simulink model "Robot_Sim_bkp2"  (R2017a)
settings: Solver=VariableStepAuto  StartTime=0.0  StopTime=Tsim  FixedStep=Ts_compute  RelTol=1e-3
values from neighbouring files (symbols this model uses):
  b = 0.1    [Model_old.m]
  g = 40    [Model_old.m]    (also in ModeloBase_OLD.m)
  Gyro_bias = 0.004    [Model_old.m]
  Kd = 0    [Model_old.m]
  Ki = 10.0    (= 10)    [Model_old.m]
  Kp = 5.0    (= 5)    [Model_old.m]
  ksi = 0.6    [Model_old.m]    (also in ModeloBase_OLD.m = 0.3)
  Ts = 0.1    [Model_old.m]    (also in ModeloBase_OLD.m; PIController.m)
  Ts_sensor = 1/50    (= 0.02)    [Model_old.m]
  Tsim = 50    [Model_old.m]    (also in ModeloBase_OLD.m = 70)
undefined symbols (not defined in the file or in its folder): Aa, Ag, Ba, Bg, Ca, Cg, DiscIntNeverNeededParam, Discrete, K_KALM_g, K_LQ, Rna, Rng, Time, W
undefined symbols (not defined in the file): Qna
libraries: simulink x13, ctrlSharedLib x2, cstblocks x2
settings Model: PauseTimes=28  NumberOfSteps=10  Creator=davi2  LastModifiedBy=marcus

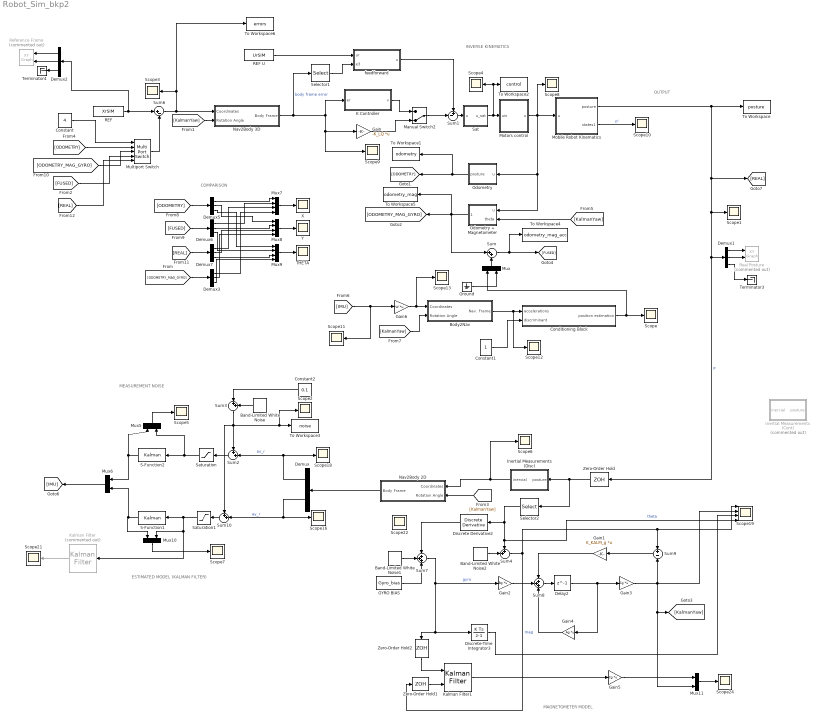
== system Robot_Sim_bkp2 ==
  note: COMPARISON
  note: OUTPUT
  note: MEASUREMENT NOISE
  note: INVERSE KINEMATICS
  note: MAGNETOMETER MODEL
  note: ESTIMATED MODEL (KALMAN FILTER)
  Band-Limited White Noise : simulink/Sources/Band-Limited White Noise  Cov=Rna^2  Ts=Ts_sensor  seed=[23341]
  Band-Limited White Noise1 : simulink/Sources/Band-Limited White Noise  Cov=0.00001  Ts=Ts_sensor  seed=[23341]
  Band-Limited White Noise2 : simulink/Sources/Band-Limited White Noise  Cov=Rng^2  Ts=Ts_sensor  seed=[23341]
  Body2Nav : Subsystem
  Conditioning Block : Subsystem
  Constant : Constant  Value=4
  Constant1 : Constant
  Constant2 : Constant  Value=0.1
  Delay2 : Delay  DelayLength=1
  Demux : Demux  Outputs=2
  Demux{1..3,5..7} (6 alike) : Demux  Outputs=3
  Discrete Derivative2 : simulink/Discrete/Discrete Derivative  gainval=1.0  ICPrevScaledInput=0.0  OutMin=[]  OutMax=[]  OutDataType=fixdt(1, 16)  OutScaling=2^-10  DoSatur=off
  Discrete-Time Integrator3 : DiscreteIntegrator  InitialConditionSetting=State (most efficient)  SampleTime=-1  ICPrevOutput=DiscIntNeverNeededParam  ICPrevScaledInput=DiscIntNeverNeededParam
  GYRO BIAS : Constant  Value=Gyro_bias
  Gain : Gain  Gain=-K_LQ  Multiplication=Matrix(K*u)
  Gain1 : Gain  Gain=K_KALM_g  Multiplication=Matrix(K*u)
  Gain2 : Gain  Gain=Bg  Multiplication=Matrix(K*u)
  Gain3 : Gain  Gain=Cg  Multiplication=Matrix(K*u)
  Gain4 : Gain  Gain=Ag  Multiplication=Matrix(K*u)
  Gain5 : Gain  Gain=Cg  Multiplication=Matrix(K*u)
  Gain6 : Gain  Gain=W  Multiplication=Matrix(K*u)
  Ground : Ground
  Inertial Measurements (Cont) : Subsystem  Commented=on
  Inertial Measurements (Disc) : Subsystem
  K Controller : Subsystem
  Kalman Filter : ctrlSharedLib/Kalman Filter  Commented=on  TimeDomain=Discrete-Time  UseCurrentEstimator=on  ModelSource=LTI State-Space Variable  ModelSourceVariable=ss(Aa,Ba,Ca,0,Ts_sensor)  A=0.95  B=1  C=1  D=0  NumberOfStates=1  NumberOfInputs=1  NumberOfOutputs=1  InitialEstimateSource=Dialog  X0=0  P0=10  UseK=off  UseGH=off  NumberOfProcessNoiseInputs=1  G=1  TimeInvariantG=on  H=0  TimeInvariantH=on  Q=Qna  TimeInvariantQ=on  R=Rna  TimeInvariantR=on  N=0  TimeInvariantN=on  AddInputPort=off  AddEnablePort=off  OutputEstimatedY=off  OutputP=off  Ts=-1
  Kalman Filter1 : ctrlSharedLib/Kalman Filter  TimeDomain=Discrete-Time  UseCurrentEstimator=on  ModelSource=LTI State-Space Variable  ModelSourceVariable=ss(Ag,Bg,Cg,0,Ts_sensor)  A=0.95  B=1  C=1  D=0  NumberOfStates=1  NumberOfInputs=1  NumberOfOutputs=1  InitialEstimateSource=Dialog  X0=0  P0=10  UseK=off  UseGH=off  NumberOfProcessNoiseInputs=1  G=1  TimeInvariantG=on  H=0  TimeInvariantH=on  Q=Qng  TimeInvariantQ=on  R=Rng  TimeInvariantR=on  N=0  TimeInvariantN=on  AddInputPort=on  AddEnablePort=off  OutputEstimatedY=off  OutputP=off  Ts=-1
  Manual Switch2 : ManualSwitch  CurrentSetting=0
  Mobile Robot Kinematics : Subsystem
  Motors control : Subsystem
  Multiport Switch : MultiPortSwitch  Inputs=4
  Mux{,5..6,10..11} (5 alike) : Mux  Inputs=2
  Mux7 : Mux
  Mux8 : Mux
  Mux9 : Mux
  Nav2Body 2D : Subsystem
  Nav2Body 3D : Subsystem
  Odometry : Subsystem
  Odometry + Magnetometer : Subsystem
  REF : FromWorkspace  VariableName=XrSIM  SampleTime=Ts  OutputAfterFinalValue=Holding final value
  REF U : FromWorkspace  VariableName=UrSIM  SampleTime=Ts  OutputAfterFinalValue=Holding final value
  Real Posture : simulink/Sinks/XY Graph  Commented=on  xmin=0  xmax=3  ymin=-0.8  ymax=1.5  st=Ts
  Reference Frame : simulink/Sinks/XY Graph  Commented=on  xmin=0  xmax=2  ymin=0  ymax=1.5  st=Ts
  S-Function1 : S-Function  FunctionName=Kalman  Parameters=Ts_sensor,A,C,Rw,Rv  SFunctionDeploymentMode=off  EnableBusSupport=off  mask{Ts=Ts_sensor, A=Aa, C=Ca, Rv=Rna, Rw=Qna}
      mask prompts: Ts "Tempo de Amostragem"; A "Matriz A"; C "Matriz C"; Rv "Covariancia da Saida"; Rw "Covariancia do Processo"
      mask DialogControl DescTextVar Tooltip: Filtro
      mask Display: disp('MyKalman')
  S-Function2 : S-Function  FunctionName=Kalman  Parameters=Ts_sensor,A,C,Rw,Rv  SFunctionDeploymentMode=off  EnableBusSupport=off  mask{Ts=Ts_sensor, A=Aa, C=Ca, Rv=Rna, Rw=Qna}
      mask prompts: Ts "Tempo de Amostragem"; A "Matriz A"; C "Matriz C"; Rv "Covariancia da Saida"; Rw "Covariancia do Processo"
      mask DialogControl DescTextVar Tooltip: Filtro
      mask Display: disp('MyKalman')
  Sat : Subsystem
  Saturation : Saturate  UpperLimit=4*9.8  LowerLimit=-4*9.8
  Saturation1 : Saturate  UpperLimit=4*9.8  LowerLimit=-4*9.8
  Scope{,1..13,16,18,21..22,24} (19 alike) : Scope
  Scope19 : Scope  NumInputPorts=4
  Selector1 : Selector  InputPortWidth=3  IndexOptions=Index vector (dialog)  Indices=3  OutputSizes=1
  Selector2 : Selector  InputPortWidth=3  IndexOptions=Index vector (dialog)  Indices=3  OutputSizes=1
  Sum : Sum  Inputs=|++
  Sum1 : Sum  Inputs=+-|
  Sum10 : Sum  Inputs=++|
  Sum2 : Sum  Inputs=++|
  Sum3 : Sum  Inputs=|++
  Sum4 : Sum  Inputs=++|
  Sum6 : Sum  Inputs=|+-
  Sum7 : Sum  Inputs=+++
  Sum8 : Sum  Inputs=+++
  Sum9 : Sum  Inputs=+-
  THETA : Scope
  Terminator3 : Terminator
  Terminator4 : Terminator
  To Workspace : ToWorkspace  VariableName=posture  SaveFormat=Timeseries  SampleTime=-1
  To Workspace1 : ToWorkspace  VariableName=odometry  SaveFormat=Timeseries  SampleTime=-1
  To Workspace2 : ToWorkspace  VariableName=control  SaveFormat=Timeseries  SampleTime=-1
  To Workspace3 : ToWorkspace  VariableName=noise  SaveFormat=Timeseries  SampleTime=-1
  To Workspace4 : ToWorkspace  VariableName=odometry_mag_acc  SaveFormat=Timeseries  SampleTime=-1
  To Workspace5 : ToWorkspace  VariableName=odometry_mag  SaveFormat=Timeseries  SampleTime=-1
  To Workspace6 : ToWorkspace  VariableName=errors  SaveFormat=Timeseries  SampleTime=-1
  X : Scope
  Y : Scope
  Zero-Order Hold : ZeroOrderHold  SampleTime=Ts_sensor
  Zero-Order Hold1 : ZeroOrderHold  SampleTime=Ts_sensor
  Zero-Order Hold2 : ZeroOrderHold  SampleTime=Ts_sensor
  feedforward : Subsystem
  wires:
  Nav2Body 3D/1(Body Frame) -> Scope9/1, Gain/1, K Controller/1(er), Selector1/1  "body frame error"
  REF U/1 -> feedforward/1(ur)
  Selector1/1 -> feedforward/2(e3)
  Motors control/1(u) -> Odometry + Magnetometer/1(u), Odometry/1(u), Mobile Robot Kinematics/1(u), Scope8/1
  Selector2/1 -> Scope19/4, Sum4/1, Discrete Derivative2/1  "theta"
  Demux1/1 -> Real Posture/1
  Demux1/2 -> Real Posture/2
  Odometry/1(posture) -> To Workspace1/1, [ODOMETRY]
  Sum1/1 -> Sat/1(u)
  Sat/1(u_sat) -> Motors control/1(uin), Scope4/1, To Workspace2/1
  Demux1/3 -> Terminator3/1
  Band-Limited White Noise2/1 -> Sum4/2
  Demux2/1 -> Reference Frame/1
  Demux2/2 -> Reference Frame/2
  Demux2/3 -> Terminator4/1
  Mobile Robot Kinematics/1(posture) -> [REAL], Zero-Order Hold/1, Demux1/1, Scope1/1, To Workspace/1  "P"
  Demux/1 -> Scope18/1, Sum2/2  "ax_r"
  Demux/2 -> Sum10/2, Scope16/1  "ay_r"
  Inertial Measurements (Disc)/1(inercial) -> Scope6/1, Nav2Body 2D/1(Coordinates)
  REF/1 -> Sum6/1, Demux2/1
  Mux5/1 -> Scope5/1
  [KalmanYaw] -> Nav2Body 2D/2(Rotation Angle)
  Odometry + Magnetometer/1(posture) -> Sum/1, To Workspace5/1, [ODOMETRY_MAG_GYRO]
  [KalmanYaw] -> Odometry + Magnetometer/2(theta)
  [ODOMETRY] -> Demux5/1
  [FUSED] -> Demux6/1
  [REAL] -> Demux7/1
  Demux5/1 -> Mux7/1
  Demux6/1 -> Mux7/2
  Demux7/1 -> Mux7/3
  Mux7/1 -> X/1
  Demux5/2 -> Mux8/1
  Demux6/2 -> Mux8/2
  Demux7/2 -> Mux8/3
  Demux5/3 -> Mux9/1
  Demux6/3 -> Mux9/2
  Demux7/3 -> Mux9/3
  Mux8/1 -> Y/1
  Mux9/1 -> THETA/1
  Mobile Robot Kinematics/2(states1) -> Scope10/1  "p'"
  Sum3/1 -> Sum10/1, Sum2/1, Scope2/1, To Workspace3/1
  Band-Limited White Noise/1 -> Sum3/2
  Constant2/1 -> Sum3/1
  Sum10/1 -> Saturation1/1
  Sum2/1 -> Saturation/1
  Saturation1/1 -> S-Function1/1, Mux10/2, Kalman Filter/1
  Saturation/1 -> S-Function2/1, Mux5/2
  Mux10/1 -> Scope7/1
  S-Function1/1 -> Mux6/2, Mux10/1
  S-Function2/1 -> Mux6/1, Mux5/1
  Band-Limited White Noise1/1 -> Sum7/2
  Discrete Derivative2/1 -> Sum7/1
  GYRO BIAS/1 -> Sum7/3
  Sum7/1 -> Gain2/1, Discrete-Time Integrator3/1, Zero-Order Hold2/1  "gyro"
  Sum4/1 -> Scope19/1, Sum9/1, Zero-Order Hold1/1  "mag"
  Sum8/1 -> Delay2/1
  Gain2/1 -> Sum8/2
  Delay2/1 -> Gain3/1, Gain4/1
  Gain4/1 -> Sum8/3
  Gain1/1 -> Sum8/1
  Gain3/1 -> Scope19/2, Mux11/2, [KalmanYaw], Sum9/2
  Sum9/1 -> Gain1/1
  Discrete-Time Integrator3/1 -> Scope19/3
  Manual Switch2/1 -> Sum1/2
  feedforward/1(u) -> Sum1/1
  Gain/1 -> Manual Switch2/2
  K Controller/1(v) -> Manual Switch2/1
  Nav2Body 2D/1(Body Frame) -> Demux/1
  [KalmanYaw] -> Nav2Body 3D/2(Rotation Angle)
  Mux6/1 -> [IMU]
  Sum6/1 -> To Workspace6/1, Scope3/1, Nav2Body 3D/1(Coordinates)
  Kalman Filter/1 -> Scope21/1
  Zero-Order Hold1/1 -> Kalman Filter1/2
  Zero-Order Hold2/1 -> Kalman Filter1/1
  Kalman Filter1/1 -> Gain5/1
  Mux11/1 -> Scope24/1
  Gain5/1 -> Mux11/1
  Zero-Order Hold/1 -> Inertial Measurements (Disc)/1(posture), Selector2/1
  [ODOMETRY_MAG_GYRO] -> Demux3/1
  Demux3/1 -> Mux7/4
  Demux3/2 -> Mux8/4
  Demux3/3 -> Mux9/4
  [ODOMETRY] -> Multiport Switch/2
  [ODOMETRY_MAG_GYRO] -> Multiport Switch/3
  [FUSED] -> Multiport Switch/4
  Multiport Switch/1 -> Sum6/2
  Constant/1 -> Multiport Switch/1
  [KalmanYaw] -> Body2Nav/2(Rotation Angle)
  Sum/1 -> To Workspace4/1, [FUSED]
  Mux/1 -> Sum/2
  Ground/1 -> Mux/2
  Constant1/1 -> Conditioning Block/2(discriminant)
  [IMU] -> Gain6/1, Scope11/1
  Conditioning Block/1(position estimation) -> Mux/1, Scope/1
  [REAL] -> Multiport Switch/5
  Body2Nav/1(Nav. Frame) -> Scope12/1, Conditioning Block/1(accelerations)
  Gain6/1 -> Scope13/1, Body2Nav/1(Coordinates)

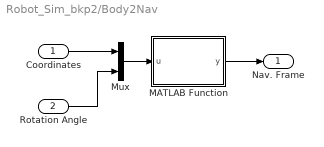
== system Robot_Sim_bkp2/Body2Nav ==
  Coordinates : Inport
  Rotation Angle : Inport  Port=2
  MATLAB Function : MATLAB Function  TreatAsAtomicUnit=on
  Mux : Mux  Inputs=2
  Nav. Frame : Outport
  wires:
  Coordinates/1 -> Mux/1
  Rotation Angle/1 -> Mux/2
  Mux/1 -> MATLAB Function/1(u)
  MATLAB Function/1(y) -> Nav. Frame/1

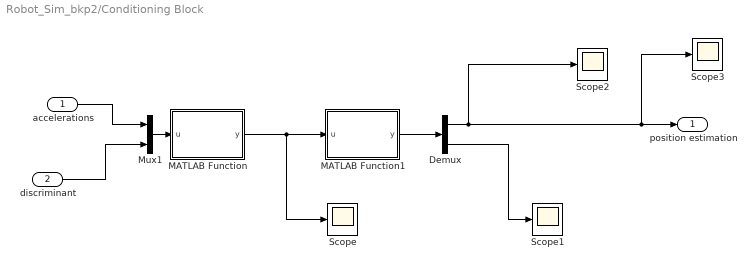
== system Robot_Sim_bkp2/Conditioning Block ==
  accelerations : Inport
  discriminant : Inport  Port=2
  Demux : Demux  Outputs=2
  MATLAB Function : MATLAB Function  TreatAsAtomicUnit=on
  MATLAB Function1 : MATLAB Function  TreatAsAtomicUnit=on
  Mux1 : Mux  Inputs=2
  Scope{,1..3} (4 alike) : Scope
  position estimation : Outport
  wires:
  Mux1/1 -> MATLAB Function/1(u)
  accelerations/1 -> Mux1/1
  MATLAB Function/1(y) -> MATLAB Function1/1(u), Scope/1
  MATLAB Function1/1(y) -> Demux/1
  discriminant/1 -> Mux1/2
  Demux/2 -> Scope1/1
  Demux/1 -> Scope3/1, position estimation/1, Scope2/1

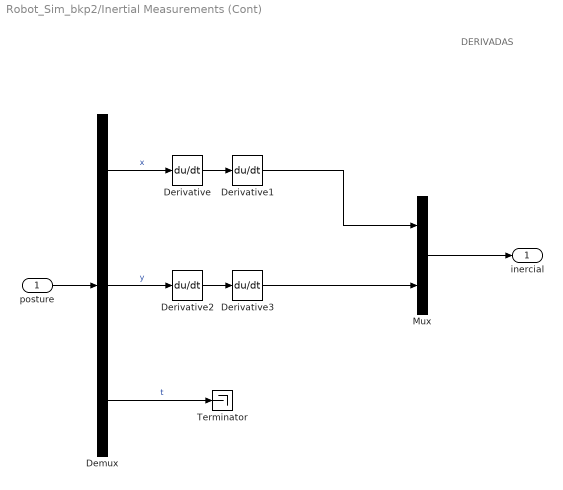
== system Robot_Sim_bkp2/Inertial Measurements (Cont) ==
  note: DERIVADAS
  posture : Inport
  Demux : Demux  Outputs=3
  Derivative{,1..3} (4 alike) : Derivative
  Mux : Mux  Inputs=2
  Terminator : Terminator
  inercial : Outport
  wires:
  posture/1 -> Demux/1
  Mux/1 -> inercial/1
  Demux/3 -> Terminator/1  "t"
  Derivative3/1 -> Mux/2
  Derivative1/1 -> Mux/1
  Demux/1 -> Derivative/1  "x"
  Demux/2 -> Derivative2/1  "y"
  Derivative/1 -> Derivative1/1
  Derivative2/1 -> Derivative3/1

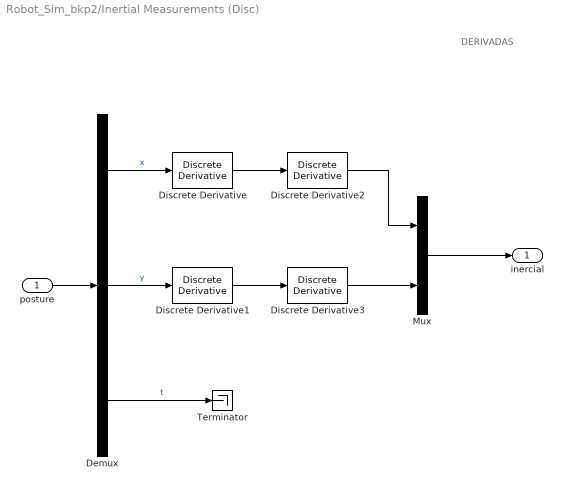
== system Robot_Sim_bkp2/Inertial Measurements (Disc) ==
  note: DERIVADAS
  posture : Inport
  Demux : Demux  Outputs=3
  Discrete Derivative{,1..3} (4 alike) : simulink/Discrete/Discrete Derivative  gainval=1.0  ICPrevScaledInput=0.0  OutMin=[]  OutMax=[]  OutDataType=fixdt(1, 16)  OutScaling=2^-10  DoSatur=off
  Mux : Mux  Inputs=2
  Terminator : Terminator
  inercial : Outport
  wires:
  posture/1 -> Demux/1
  Mux/1 -> inercial/1
  Demux/3 -> Terminator/1  "t"
  Discrete Derivative1/1 -> Discrete Derivative3/1
  Discrete Derivative3/1 -> Mux/2
  Discrete Derivative2/1 -> Mux/1
  Discrete Derivative/1 -> Discrete Derivative2/1
  Demux/1 -> Discrete Derivative/1  "x"
  Demux/2 -> Discrete Derivative1/1  "y"

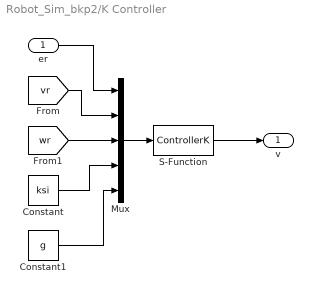
== system Robot_Sim_bkp2/K Controller ==
  er : Inport
  Constant : Constant  Value=ksi
  Constant1 : Constant  Value=g
  Mux : Mux  Inputs=5
  S-Function : S-Function  FunctionName=ControllerK  Parameters=Ts  SFunctionDeploymentMode=off  EnableBusSupport=off
  v : Outport
  wires:
  er/1 -> Mux/1
  [vr] -> Mux/2
  [wr] -> Mux/3
  Constant/1 -> Mux/4
  Constant1/1 -> Mux/5
  Mux/1 -> S-Function/1
  S-Function/1 -> v/1

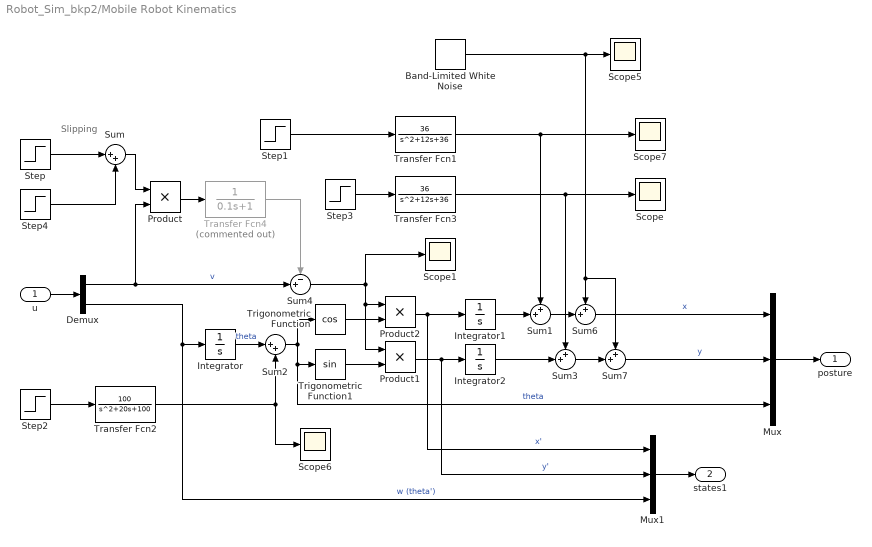
== system Robot_Sim_bkp2/Mobile Robot Kinematics ==
  note: Slipping
  u : Inport
  Band-Limited White Noise : simulink/Sources/Band-Limited White Noise  Cov=0  Ts=Ts_sensor  seed=[23341]
  Demux : Demux  Outputs=2
  Integrator : Integrator
  Integrator1 : Integrator
  Integrator2 : Integrator
  Mux : Mux  Inputs=3
  Mux1 : Mux  Inputs=3
  Product : Product
  Product1 : Product
  Product2 : Product
  Scope{,1,5..7} (5 alike) : Scope
  Step : Step  Time=25  SampleTime=0
  Step1 : Step  Time=Tsim/2  After=0.5  SampleTime=0
  Step2 : Step  Time=Tsim/4  After=0.5  SampleTime=0
  Step3 : Step  Time=Tsim/4  After=0.5  SampleTime=0
  Step4 : Step  Time=27  After=-1  SampleTime=0
  Sum : Sum  Inputs=|++
  Sum{1,3,6..7} (4 alike) : Sum  Inputs=++|
  Sum2 : Sum  Inputs=|++
  Sum4 : Sum  Inputs=-+|
  Transfer Fcn1 : TransferFcn  Numerator=36  Denominator=[1 12 36]
  Transfer Fcn2 : TransferFcn  Numerator=100  Denominator=[1 20 100]
  Transfer Fcn3 : TransferFcn  Numerator=36  Denominator=[1 12 36]
  Transfer Fcn4 : TransferFcn  Commented=on  Numerator=1  Denominator=[0.1 1]
  Trigonometric Function : Trigonometry  Operator=cos
  Trigonometric Function1 : Trigonometry
  posture : Outport
  states1 : Outport  Port=2
  wires:
  u/1 -> Demux/1
  Demux/2 -> Integrator/1, Mux1/3  "w (theta')"
  Trigonometric Function/1 -> Product2/2
  Demux/1 -> Sum4/2, Product/2  "v"
  Trigonometric Function1/1 -> Product1/2
  Mux/1 -> posture/1
  Step2/1 -> Transfer Fcn2/1
  Integrator/1 -> Sum2/1  "theta"
  Sum2/1 -> Mux/3, Trigonometric Function1/1, Trigonometric Function/1  "theta"
  Transfer Fcn2/1 -> Sum2/2, Scope6/1
  Product1/1 -> Mux1/2, Integrator2/1  "y'"
  Product2/1 -> Mux1/1, Integrator1/1  "x'"
  Step1/1 -> Transfer Fcn1/1
  Step3/1 -> Transfer Fcn3/1
  Integrator1/1 -> Sum1/2
  Integrator2/1 -> Sum3/2
  Transfer Fcn3/1 -> Sum3/1, Scope/1
  Transfer Fcn1/1 -> Scope7/1, Sum1/1
  Step/1 -> Sum/1
  Step4/1 -> Sum/2
  Sum/1 -> Product/1
  Sum4/1 -> Scope1/1, Product1/1, Product2/1
  Product/1 -> Transfer Fcn4/1
  Transfer Fcn4/1 -> Sum4/1
  Mux1/1 -> states1/1
  Sum1/1 -> Sum6/2
  Sum3/1 -> Sum7/2
  Sum7/1 -> Mux/2  "y"
  Sum6/1 -> Mux/1  "x"
  Band-Limited White Noise/1 -> Scope5/1, Sum7/1, Sum6/1

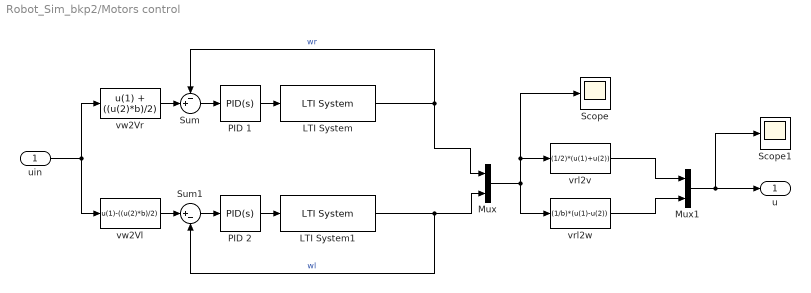
== system Robot_Sim_bkp2/Motors control ==
  uin : Inport
  LTI System : cstblocks/LTI System  sys=HMotor  IC=[]
  LTI System1 : cstblocks/LTI System  sys=HMotor  IC=[]
  Mux : Mux  Inputs=2
  Mux1 : Mux  Inputs=2
  PID 1 : simulink/Continuous/PID Controller  Controller=PID  TimeDomain=Continuous-time  SampleTime=-1  IntegratorMethod=Forward Euler  FilterMethod=Forward Euler  Form=Parallel  UseFilter=on  ControllerParametersSource=internal  P=Kp  I=Ki  D=Kd  N=100  InitialConditionSource=internal  InitialConditionForIntegrator=0  InitialConditionForFilter=0  ExternalReset=none  LimitOutput=off  UpperSaturationLimit=inf  LowerSaturationLimit=-inf  LinearizeAsGain=on  AntiWindupMode=none  Kb=1  TrackingMode=off  Kt=1  PParamMin=[]  PParamMax=[]  IParamMin=[]  IParamMax=[]  DParamMin=[]  DParamMax=[]  NParamMin=[]  NParamMax=[]  KbParamMin=[]  KbParamMax=[]  KtParamMin=[]  KtParamMax=[]  POutMin=[]  POutMax=[]  IOutMin=[]  IOutMax=[]  DOutMin=[]  DOutMax=[]  NOutMin=[]  NOutMax=[]  KbOutMin=[]  KbOutMax=[]  KtOutMin=[]  KtOutMax=[]  IntegratorOutMin=[]  IntegratorOutMax=[]  FilterOutMin=[]  FilterOutMax=[]  SumOutMin=[]  SumOutMax=[]  SumI1OutMin=[]  SumI1OutMax=[]  SumI2OutMin=[]  SumI2OutMax=[]  SumI3OutMin=[]  SumI3OutMax=[]  SumDOutMin=[]  SumDOutMax=[]  SaturationOutMin=[]  SaturationOutMax=[]  IntegratorContinuousStateAttributes=''  IntegratorStateMustResolveToSignalObject=off  IntegratorRTWStateStorageClass=Auto  FilterContinuousStateAttributes=''  FilterStateMustResolveToSignalObject=off  FilterRTWStateStorageClass=Auto  DifferentiatorICPrevScaledInput=0  DifferentiatorOutMin=[]  DifferentiatorOutMax=[]  InitialConditionSetting=State (most efficient)
  PID 2 : simulink/Continuous/PID Controller  Controller=PID  TimeDomain=Continuous-time  SampleTime=-1  IntegratorMethod=Forward Euler  FilterMethod=Forward Euler  Form=Parallel  UseFilter=on  ControllerParametersSource=internal  P=Kp  I=Ki  D=Kd  N=100  InitialConditionSource=internal  InitialConditionForIntegrator=0  InitialConditionForFilter=0  ExternalReset=none  LimitOutput=off  UpperSaturationLimit=inf  LowerSaturationLimit=-inf  LinearizeAsGain=on  AntiWindupMode=none  Kb=1  TrackingMode=off  Kt=1  PParamMin=[]  PParamMax=[]  IParamMin=[]  IParamMax=[]  DParamMin=[]  DParamMax=[]  NParamMin=[]  NParamMax=[]  KbParamMin=[]  KbParamMax=[]  KtParamMin=[]  KtParamMax=[]  POutMin=[]  POutMax=[]  IOutMin=[]  IOutMax=[]  DOutMin=[]  DOutMax=[]  NOutMin=[]  NOutMax=[]  KbOutMin=[]  KbOutMax=[]  KtOutMin=[]  KtOutMax=[]  IntegratorOutMin=[]  IntegratorOutMax=[]  FilterOutMin=[]  FilterOutMax=[]  SumOutMin=[]  SumOutMax=[]  SumI1OutMin=[]  SumI1OutMax=[]  SumI2OutMin=[]  SumI2OutMax=[]  SumI3OutMin=[]  SumI3OutMax=[]  SumDOutMin=[]  SumDOutMax=[]  SaturationOutMin=[]  SaturationOutMax=[]  IntegratorContinuousStateAttributes=''  IntegratorStateMustResolveToSignalObject=off  IntegratorRTWStateStorageClass=Auto  FilterContinuousStateAttributes=''  FilterStateMustResolveToSignalObject=off  FilterRTWStateStorageClass=Auto  DifferentiatorICPrevScaledInput=0  DifferentiatorOutMin=[]  DifferentiatorOutMax=[]  InitialConditionSetting=State (most efficient)
  Scope : Scope
  Scope1 : Scope
  Sum : Sum  Inputs=-+|
  Sum1 : Sum  Inputs=|+-
  vrl2v : Fcn  Expr=(1/2)*(u(1)+u(2))
  vrl2w : Fcn  Expr=(1/b)*(u(1)-u(2))
  vw2Vl : Fcn  Expr=u(1)-((u(2)*b)/2)
  vw2Vr : Fcn  Expr=u(1) + ((u(2)*b)/2)
  u : Outport
  wires:
  LTI System1/1 -> Mux/2, Sum1/2  "wl"
  vw2Vl/1 -> Sum1/1
  Sum1/1 -> PID 2/1
  PID 2/1 -> LTI System1/1
  Sum/1 -> PID 1/1
  PID 1/1 -> LTI System/1
  LTI System/1 -> Mux/1, Sum/1  "wr"
  uin/1 -> vw2Vl/1, vw2Vr/1
  Mux/1 -> vrl2w/1, Scope/1, vrl2v/1
  Mux1/1 -> Scope1/1, u/1
  vrl2v/1 -> Mux1/1
  vrl2w/1 -> Mux1/2
  vw2Vr/1 -> Sum/2

== system Robot_Sim_bkp2/Nav2Body 2D ==
  Coordinates : Inport
  Rotation Angle : Inport  Port=2
  MATLAB Function : MATLAB Function  TreatAsAtomicUnit=on
  Mux : Mux  Inputs=2
  Body Frame : Outport
  wires:
  Coordinates/1 -> Mux/1
  Rotation Angle/1 -> Mux/2
  Mux/1 -> MATLAB Function/1(u)
  MATLAB Function/1(y) -> Body Frame/1

== system Robot_Sim_bkp2/Nav2Body 3D ==
  Coordinates : Inport
  Rotation Angle : Inport  Port=2
  MATLAB Function : MATLAB Function  TreatAsAtomicUnit=on
  Mux : Mux  Inputs=2
  Body Frame : Outport
  wires:
  Coordinates/1 -> Mux/1
  Rotation Angle/1 -> Mux/2
  Mux/1 -> MATLAB Function/1(u)
  MATLAB Function/1(y) -> Body Frame/1

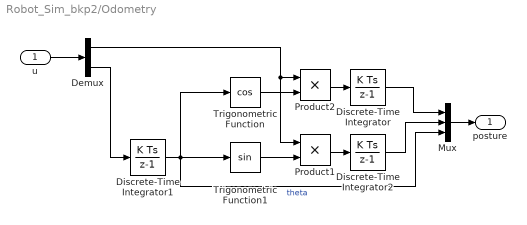
== system Robot_Sim_bkp2/Odometry ==
  u : Inport
  Demux : Demux  Outputs=2
  Discrete-Time Integrator : DiscreteIntegrator  InitialConditionSetting=State (most efficient)  SampleTime=Ts  ICPrevOutput=DiscIntNeverNeededParam  ICPrevScaledInput=DiscIntNeverNeededParam
  Discrete-Time Integrator1 : DiscreteIntegrator  InitialConditionSetting=State (most efficient)  SampleTime=Ts  ICPrevOutput=DiscIntNeverNeededParam  ICPrevScaledInput=DiscIntNeverNeededParam
  Discrete-Time Integrator2 : DiscreteIntegrator  InitialConditionSetting=State (most efficient)  SampleTime=Ts  ICPrevOutput=DiscIntNeverNeededParam  ICPrevScaledInput=DiscIntNeverNeededParam
  Mux : Mux  Inputs=3
  Product1 : Product
  Product2 : Product
  Trigonometric Function : Trigonometry  Operator=cos
  Trigonometric Function1 : Trigonometry
  posture : Outport
  wires:
  u/1 -> Demux/1
  Demux/2 -> Discrete-Time Integrator1/1
  Trigonometric Function/1 -> Product2/2
  Demux/1 -> Product1/1, Product2/1
  Product2/1 -> Discrete-Time Integrator/1
  Trigonometric Function1/1 -> Product1/2
  Product1/1 -> Discrete-Time Integrator2/1
  Discrete-Time Integrator/1 -> Mux/1
  Discrete-Time Integrator2/1 -> Mux/2
  Mux/1 -> posture/1
  Discrete-Time Integrator1/1 -> Mux/3, Trigonometric Function1/1, Trigonometric Function/1  "theta"

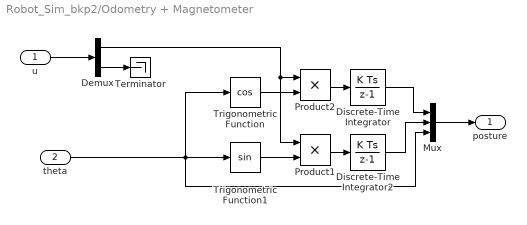
== system Robot_Sim_bkp2/Odometry + Magnetometer ==
  u : Inport
  theta : Inport  Port=2
  Demux : Demux  Outputs=2
  Discrete-Time Integrator : DiscreteIntegrator  InitialConditionSetting=State (most efficient)  SampleTime=Ts  ICPrevOutput=DiscIntNeverNeededParam  ICPrevScaledInput=DiscIntNeverNeededParam
  Discrete-Time Integrator2 : DiscreteIntegrator  InitialConditionSetting=State (most efficient)  SampleTime=Ts  ICPrevOutput=DiscIntNeverNeededParam  ICPrevScaledInput=DiscIntNeverNeededParam
  Mux : Mux  Inputs=3
  Product1 : Product
  Product2 : Product
  Terminator : Terminator
  Trigonometric Function : Trigonometry  Operator=cos
  Trigonometric Function1 : Trigonometry
  posture : Outport
  wires:
  u/1 -> Demux/1
  Trigonometric Function/1 -> Product2/2
  Demux/1 -> Product1/1, Product2/1
  Product2/1 -> Discrete-Time Integrator/1
  Trigonometric Function1/1 -> Product1/2
  Product1/1 -> Discrete-Time Integrator2/1
  Discrete-Time Integrator/1 -> Mux/1
  Discrete-Time Integrator2/1 -> Mux/2
  Mux/1 -> posture/1
  Demux/2 -> Terminator/1
  theta/1 -> Mux/3, Trigonometric Function/1, Trigonometric Function1/1

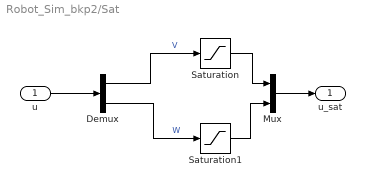
== system Robot_Sim_bkp2/Sat ==
  u : Inport
  Demux : Demux  Outputs=2
  Mux : Mux  Inputs=2
  Saturation : Saturate  UpperLimit=0.4  LowerLimit=0
  Saturation1 : Saturate  UpperLimit=0.8  LowerLimit=-0.8
  u_sat : Outport
  wires:
  Demux/2 -> Saturation1/1  "W"
  Demux/1 -> Saturation/1  "V"
  u/1 -> Demux/1
  Saturation/1 -> Mux/1
  Saturation1/1 -> Mux/2
  Mux/1 -> u_sat/1

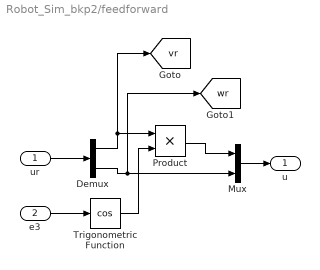
== system Robot_Sim_bkp2/feedforward ==
  ur : Inport
  e3 : Inport  Port=2
  Demux : Demux  Outputs=2
  Mux : Mux  Inputs=2
  Product : Product
  Trigonometric Function : Trigonometry  Operator=cos
  u : Outport
  tag scope: vr=global, wr=global
  wires:
  e3/1 -> Trigonometric Function/1
  ur/1 -> Demux/1
  Demux/1 -> [vr], Product/1
  Trigonometric Function/1 -> Product/2
  Product/1 -> Mux/1
  Demux/2 -> [wr], Mux/2
  Mux/1 -> u/1

== matlab function Robot_Sim_bkp2/Nav2Body 3D/MATLAB Function ==
  data: u input; y output
function y = fcn(u)
xin = u(1);
yin = u(2);
thetain = u(3);
roation = u(4);

M = [cos(roation) sin(roation) 0;
     -sin(roation) cos(roation) 0;
     0 0 1];
 
y = M*[u(1) u(2) u(3)]';

== matlab function Robot_Sim_bkp2/Nav2Body 2D/MATLAB Function ==
  data: u input; y output
function y = fcn(u)
xin = u(1);
yin = u(2);
rotation = u(3);

M = [cos(rotation) sin(rotation);
     -sin(rotation) cos(rotation)];
 
y = M*[u(1) u(2)]';

== matlab function Robot_Sim_bkp2/Conditioning Block/MATLAB Function ==
  data: u input; y output
function y = fcn(u)
%u(1:2) = x,y
%u(3) = disc
out = u(1:2);
if u(1) < u(3)
   out(1) = 0;
end
if u(2) < u(3)
    out(2) = 0;
end
y = out;

== matlab function Robot_Sim_bkp2/Conditioning Block/MATLAB Function1 ==
  data: u input; y output
function y = fcn(u)
Ts_sensor = 1/50;
persistent buffer k vx vy px py;
N = 5;
if isempty(buffer)
    buffer = zeros(N,length(u));
    vx = 0;vy=0;
    px = 0;py=0;
end
if isempty(k)
    k = 1;
end

buffer(k,:) = u;
k = k+1;
if(k==N+1)
    k=1;
end


soma = sum(buffer);
if(soma(1) == 0)
    vx = 0;
end

if(soma(2) == 0)
    vy = 0;
end

ax = u(1);
ay = u(2);

vx = vx + ax*Ts_sensor;
vy = vy + ay*Ts_sensor;

px = px + vx*Ts_sensor;
py = py + vy*Ts_sensor;




y = [px py vx vy]';

== matlab function Robot_Sim_bkp2/Body2Nav/MATLAB Function ==
  data: u input; y output
function y = fcn(u)
xin = u(1);
yin = u(2);
rotation = u(3);

M = [cos(rotation) -sin(rotation);
     sin(rotation) cos(rotation)];
 
y = M*[u(1) u(2)]';
